simulink model "siulink2"  (R2016a)
settings: Solver=VariableStepAuto  StartTime=0.0  StopTime=10.0  RelTol=1e-3
settings Model: Creator=hdt04  LastModifiedBy=hdt04

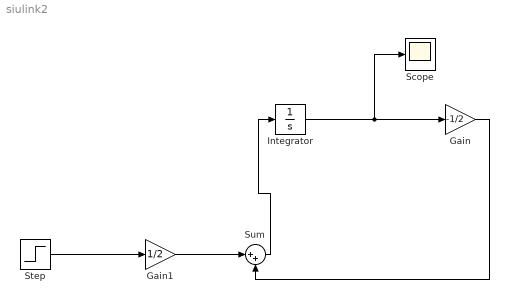
== system siulink2 ==
  Gain : Gain  Gain=-1/2
  Gain1 : Gain  Gain=1/2
  Integrator : Integrator
  Scope : Scope
  Step : Step  SampleTime=0
  Sum : Sum  Inputs=|++
  wires:
  Step/1 -> Gain1/1
  Gain1/1 -> Sum/1
  Sum/1 -> Integrator/1
  Gain/1 -> Sum/2
  Integrator/1 -> Scope/1, Gain/1
